simulink model "calcul_SA_SR"  (R2024b)
settings: Solver=FixedStepDiscrete  StartTime=0.0  StopTime=10.0  FixedStep=Ts  RelTol=1e-3
values from neighbouring files (symbols this model uses):
  epsilon = 0.1    [main_data_vehicle.m]
  lf = L*fr    (= 0.775)    [main_data_vehicle.m]
  lr = L-lf    (= 0.775)    [main_data_vehicle.m]
  Re = 0.228    [main_data_vehicle.m]
settings Model: Creator=marti  LastModifiedBy=marti

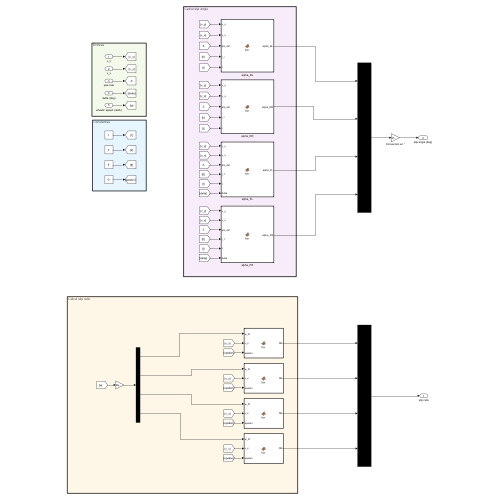
[thumbnail: Simulink's stored preview of the top-level diagram]
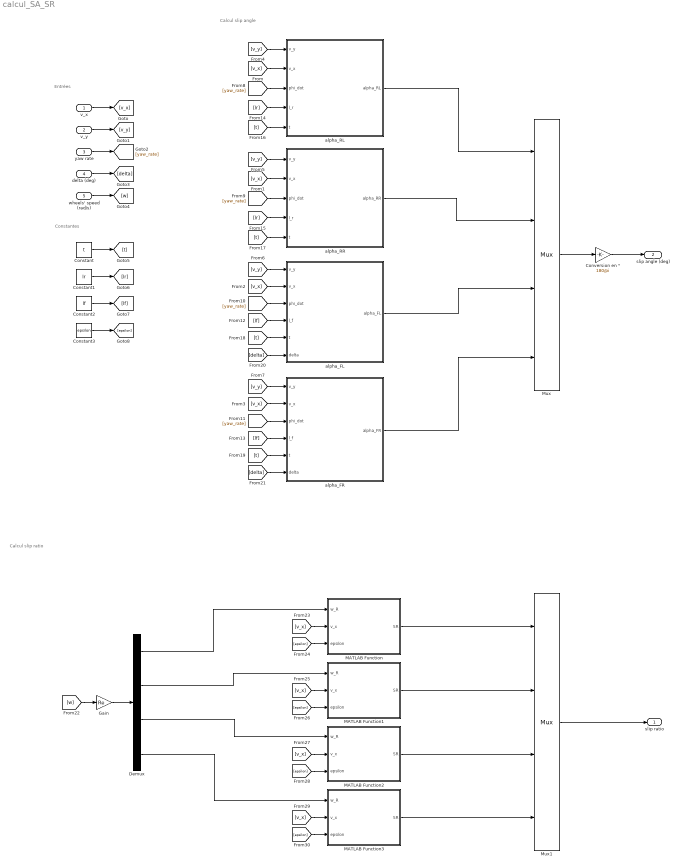
== system calcul_SA_SR ==
  note: Calcul slip ratio
  note: Calcul slip angle
  note: Constantes
  note: Entrées
  v_x : Inport
  v_y : Inport  Port=2
  yaw rate : Inport  Port=3
  delta (deg) : Inport  Port=4
  wheels' speed (rad/s) : Inport  Port=5
  Constant : Constant  Value=t
  Constant1 : Constant  Value=lr
  Constant2 : Constant  Value=lf
  Constant3 : Constant  Value=epsilon
  Conversion en ° : Gain  Gain=180/pi
  Demux : Demux
  Gain : Gain  Gain=Re
  MATLAB Function : MATLAB Function  TreatAsAtomicUnit=on
  MATLAB Function1 : MATLAB Function  TreatAsAtomicUnit=on
  MATLAB Function2 : MATLAB Function  TreatAsAtomicUnit=on
  MATLAB Function3 : MATLAB Function  TreatAsAtomicUnit=on
  Mux : Mux
  Mux1 : Mux
  alpha_FL : MATLAB Function  TreatAsAtomicUnit=on
  alpha_FR : MATLAB Function  TreatAsAtomicUnit=on
  alpha_RL : MATLAB Function  TreatAsAtomicUnit=on
  alpha_RR : MATLAB Function  TreatAsAtomicUnit=on
  slip ratio : Outport
  slip angle (deg) : Outport  Port=2
  wires:
  v_x/1 -> [v_x]
  v_y/1 -> [v_y]
  yaw rate/1 -> [yaw_rate]
  delta (deg)/1 -> [delta]
  wheels' speed (rad/s)/1 -> [w]
  Constant/1 -> [t]
  Constant1/1 -> [lr]
  Constant2/1 -> [lf]
  [v_x] -> alpha_RL/2(v_x)
  [v_x] -> alpha_RR/2(v_x)
  [v_x] -> alpha_FL/2(v_x)
  [v_x] -> alpha_FR/2(v_x)
  [v_y] -> alpha_RL/1(v_y)
  [v_y] -> alpha_RR/1(v_y)
  [v_y] -> alpha_FL/1(v_y)
  [v_y] -> alpha_FR/1(v_y)
  [yaw_rate] -> alpha_RL/3(phi_dot)
  [yaw_rate] -> alpha_RR/3(phi_dot)
  [yaw_rate] -> alpha_FL/3(phi_dot)
  [yaw_rate] -> alpha_FR/3(phi_dot)
  [lf] -> alpha_FL/4(l_f)
  [lf] -> alpha_FR/4(l_f)
  [lr] -> alpha_RL/4(l_r)
  [lr] -> alpha_RR/4(l_r)
  [t] -> alpha_RL/5(t)
  [t] -> alpha_RR/5(t)
  [t] -> alpha_FL/5(t)
  [t] -> alpha_FR/5(t)
  [delta] -> alpha_FL/6(delta)
  [delta] -> alpha_FR/6(delta)
  alpha_RR/1(alpha_RR) -> Mux/2
  alpha_FL/1(alpha_FL) -> Mux/3
  alpha_FR/1(alpha_FR) -> Mux/4
  alpha_RL/1(alpha_RL) -> Mux/1
  Mux/1 -> Conversion en °/1
  Conversion en °/1 -> slip angle (deg)/1
  [w] -> Gain/1
  Gain/1 -> Demux/1
  [v_x] -> MATLAB Function/2(v_x)
  Constant3/1 -> [epsilon]
  [epsilon] -> MATLAB Function/3(epsilon)
  [v_x] -> MATLAB Function1/2(v_x)
  [epsilon] -> MATLAB Function1/3(epsilon)
  [v_x] -> MATLAB Function2/2(v_x)
  [epsilon] -> MATLAB Function2/3(epsilon)
  [epsilon] -> MATLAB Function3/3(epsilon)
  [v_x] -> MATLAB Function3/2(v_x)
  Demux/2 -> MATLAB Function1/1(w_R)
  Demux/3 -> MATLAB Function2/1(w_R)
  Demux/1 -> MATLAB Function/1(w_R)
  Demux/4 -> MATLAB Function3/1(w_R)
  MATLAB Function1/1(SR) -> Mux1/2
  MATLAB Function2/1(SR) -> Mux1/3
  MATLAB Function/1(SR) -> Mux1/1
  MATLAB Function3/1(SR) -> Mux1/4
  Mux1/1 -> slip ratio/1

== matlab function calcul_SA_SR/alpha_RR ==
  data: v_y input; alpha_RR output; v_x input; phi_dot input; l_r input; t input
function alpha_RR = fcn(v_y,v_x,phi_dot,l_r,t)

alpha_RR = (v_y-phi_dot*l_r)/(v_x+phi_dot*t/2);
end

== matlab function calcul_SA_SR/alpha_RL ==
  data: v_y input; alpha_RL output; v_x input; phi_dot input; l_r input; t input
function alpha_RL = fcn(v_y,v_x,phi_dot,l_r,t)

alpha_RL = (v_y-phi_dot*l_r)/(v_x-phi_dot*t/2);
end

== matlab function calcul_SA_SR/alpha_FL ==
  data: v_y input; alpha_FL output; v_x input; phi_dot input; l_f input; t input; delta input
function alpha_FL = fcn(v_y,v_x,phi_dot,l_f,t,delta)

alpha_FL = (v_y+phi_dot*l_f)/(v_x-phi_dot*t/2) - delta*pi/180;
end

== matlab function calcul_SA_SR/alpha_FR ==
  data: v_y input; alpha_FR output; v_x input; phi_dot input; l_f input; t input; delta input
function alpha_FR = fcn(v_y,v_x,phi_dot,l_f,t,delta)

alpha_FR = (v_y+phi_dot*l_f)/(v_x+phi_dot*t/2) - delta*pi/180;
end

== matlab function calcul_SA_SR/MATLAB Function ==
  data: w_R input; SR output; v_x input; epsilon input
function SR = fcn(w_R,v_x,epsilon)

SR=(w_R-v_x)/(v_x+epsilon);

== matlab function calcul_SA_SR/MATLAB Function1 ==
  data: w_R input; SR output; v_x input; epsilon input
function SR = fcn(w_R,v_x,epsilon)

SR=(w_R-v_x)/(v_x+epsilon);

== matlab function calcul_SA_SR/MATLAB Function2 ==
  data: w_R input; SR output; v_x input; epsilon input
function SR = fcn(w_R,v_x,epsilon)

SR=(w_R-v_x)/(v_x+epsilon);

== matlab function calcul_SA_SR/MATLAB Function3 ==
  data: w_R input; SR output; v_x input; epsilon input
function SR = fcn(w_R,v_x,epsilon)

SR=(w_R-v_x)/(v_x+epsilon);
